simulink model "OpenFAST_ROSCO_FFP"  (R2021b)
settings: Solver=ode4  StartTime=0.0  StopTime=TMax  FixedStep=DT  MaxStep=DT  RelTol=1e-3  EnableMultiTasking=on
values from neighbouring files (symbols this model uses):
  P = ReadWrite_FAST(fast)    [RunExample_Simulink.m]
undefined symbols (not defined in the file or in its folder): F, GetFASTPar, OutList, R, simu, strmatch
libraries: simulink x1
settings Model: Creator=bjonkman  LastModifiedBy=david
settings SolverCC: AlgebraicLoopSolver=TrustRegion
settings DataIOCC: LimitDataPoints=on  SaveFormat=Array  SignalLoggingSaveFormat=ModelDataLogs  SaveOutput=off  SaveTime=off  ReturnWorkspaceOutputs=off  SignalLoggingName=sigsOut
settings OptimizationCC: ExpressionDepthLimit=2147483647  LifeSpan=inf
settings DebuggingCC: SaveWithParameterizedLinksMsg=none  UnderspecifiedInitializationDetection=Classic  MergeDetectMultiDrivingBlocksExec=none  SignalResolutionControl=TryResolveAllWithWarning  MultiTaskDSMMsg=warning  MultiTaskCondExecSysMsg=none  FcnCallInpInsideContextMsg=warning  StateNameClashWarn=warning  SFUnexpectedBacktrackingDiag=warning  SFNoUnconditionalDefaultTransitionDiag=warning  SFExecutionAtInitializationDiag=none  SFMachineParentedDataDiag=warning  ArithmeticOperatorsInVariantConditions=warning
settings HardwareCC: ProdBitPerPointer=32  ProdBitPerSizeT=32  ProdBitPerPtrDiffT=32  ProdLargestAtomicFloat=None  ProdIntDivRoundTo=Undefined  ProdEndianess=Unspecified  ProdWordSize=32  ProdHWDeviceType=32-bit Generic  TargetUnknown=on
settings ModelReferenceCC: PropagateSignalLabelsOutOfModel=off
settings SFSimCC: SimUseLocalCustomCode=off  CustomCodeUndefinedFunction=UseInterfaceOnly
settings RTWCC: RTWUseLocalCustomCode=off
settings CodeAppCC: StateflowObjectComments=on
settings GRTTargetCC: TargetLangStandard=C89/C90 (ANSI)  CombineOutputUpdateFcns=off  GRTInterface=on
settings ConfigComp: CovMetricSettings=dw  CovSaveCumulativeToWorkspaceVar=on  CovSaveSingleToWorkspaceVar=on  CovExternalEMLEnable=off

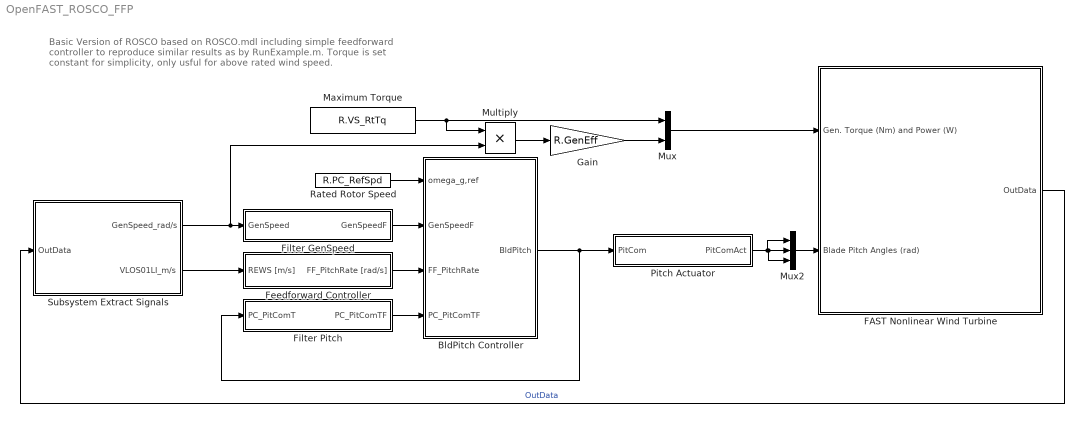
== system OpenFAST_ROSCO_FFP ==
  note: Basic Version of ROSCO based on ROSCO.mdl including simple feedforward controller to reproduce similar results as by RunExample.m.
      | Torque is set constant for simplicity, only usful for above rated wind speed.
  "  FAST Nonlinear Wind Turbine" : Subsystem  mask(FAST Nonlinear Wind Turbine){}
      mask help: This block contains the FAST S-Function.
      mask init:
      | clear FAST_SFunc
  BldPitch Controller : Subsystem
  Feedforward Controller : Subsystem
  Filter GenSpeed : Subsystem
  Filter Pitch : Subsystem
  Gain : Gain  Gain=R.GenEff
  Maximum Torque : Constant  Value=R.VS_RtTq
  Multiply : Product
  Mux : Mux  Inputs=2
  Mux2 : Mux  Inputs=3
  Pitch Actuator : Subsystem
  Rated Rotor Speed : Constant  Value=R.PC_RefSpd
  Subsystem Extract Signals : Subsystem
  wires:
  Mux2/1 -> "  FAST Nonlinear Wind Turbine"/2(Blade Pitch Angles (rad))
  BldPitch Controller/1(BldPitch) -> Filter Pitch/1(PC_PitComT), Pitch Actuator/1(PitCom)
  Rated Rotor Speed/1 -> BldPitch Controller/1(omega_g,ref)
  Subsystem Extract Signals/1(GenSpeed_rad/s) -> Multiply/2, Filter GenSpeed/1(GenSpeed)
  Maximum Torque/1 -> Mux/1, Multiply/1
  Filter GenSpeed/1(GenSpeedF) -> BldPitch Controller/2(GenSpeedF)
  Gain/1 -> Mux/2
  Mux/1 -> "  FAST Nonlinear Wind Turbine"/1(Gen. Torque (Nm) and Power (W))
  Multiply/1 -> Gain/1
  "  FAST Nonlinear Wind Turbine"/1(OutData) -> Subsystem Extract Signals/1(OutData)  "OutData"
  Filter Pitch/1(PC_PitComTF) -> BldPitch Controller/4(PC_PitComTF)
  Pitch Actuator/1(PitComAct) -> Mux2/1, Mux2/3, Mux2/2
  Feedforward Controller/1(FF_PitchRate [rad/s]) -> BldPitch Controller/3(FF_PitchRate)
  Subsystem Extract Signals/2(VLOS01LI_m/s) -> Feedforward Controller/1(REWS [m/s])

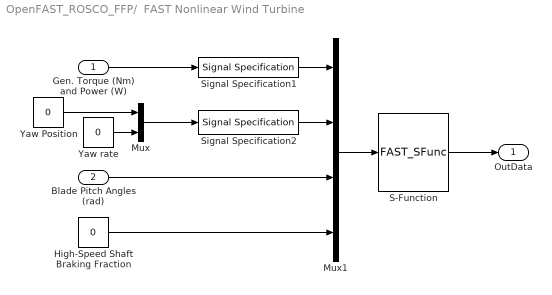
== system OpenFAST_ROSCO_FFP/  FAST Nonlinear Wind Turbine ==
  Gen. Torque (Nm) and Power (W) : Inport
  Blade Pitch Angles (rad) : Inport  Port=2
  High-Speed Shaft Braking Fraction : Constant  Value=0
  Mux : Mux  Inputs=2
  Mux1 : Mux
  S-Function : S-Function  FunctionName=FAST_SFunc  Parameters=FAST_InputFileName, TMax, 0  SFunctionDeploymentMode=off  EnableBusSupport=off
  Signal Specification1 : SignalSpecification  OutDataTypeStr=double  Dimensions=2
  Signal Specification2 : SignalSpecification  OutDataTypeStr=double  Dimensions=2
  Yaw Position : Constant  Value=0
  Yaw rate : Constant  Value=0
  OutData : Outport
  wires:
  Gen. Torque (Nm) and Power (W)/1 -> Signal Specification1/1
  S-Function/1 -> OutData/1
  Mux1/1 -> S-Function/1
  Blade Pitch Angles (rad)/1 -> Mux1/3
  Signal Specification1/1 -> Mux1/1
  Signal Specification2/1 -> Mux1/2
  High-Speed Shaft Braking Fraction/1 -> Mux1/4
  Yaw rate/1 -> Mux/2
  Mux/1 -> Signal Specification2/1
  Yaw Position/1 -> Mux/1

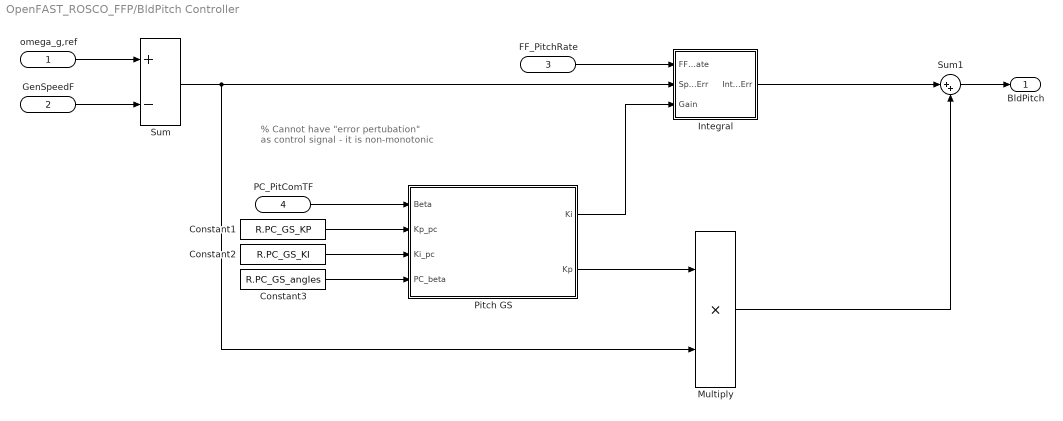
== system OpenFAST_ROSCO_FFP/BldPitch Controller ==
  note: % Cannot have "error pertubation" as control signal
      | - it is non-monotonic
  omega_g,ref : Inport
  GenSpeedF : Inport  Port=2
  FF_PitchRate : Inport  Port=3
  PC_PitComTF : Inport  Port=4
  Constant1 : Constant  Value=R.PC_GS_KP
  Constant2 : Constant  Value=R.PC_GS_KI
  Constant3 : Constant  Value=R.PC_GS_angles
  Integral : Subsystem
  Multiply : Product
  Pitch GS : MATLAB Function  TreatAsAtomicUnit=on
  Sum : Sum  Inputs=+-
  Sum1 : Sum  Inputs=|++
  BldPitch : Outport  VectorParamsAs1DForOutWhenUnconnected=off
  wires:
  Pitch GS/1(Ki) -> Integral/3(Gain)
  omega_g,ref/1 -> Sum/1
  GenSpeedF/1 -> Sum/2
  Constant1/1 -> Pitch GS/2(Kp_pc)
  Constant2/1 -> Pitch GS/3(Ki_pc)
  Constant3/1 -> Pitch GS/4(PC_beta)
  Sum/1 -> Multiply/2, Integral/2(SpeedErr)
  Multiply/1 -> Sum1/2
  Integral/1(IntSpdErr) -> Sum1/1
  Sum1/1 -> BldPitch/1
  PC_PitComTF/1 -> Pitch GS/1(Beta)
  FF_PitchRate/1 -> Integral/1(FF_PitchRate)
  Pitch GS/2(Kp) -> Multiply/1

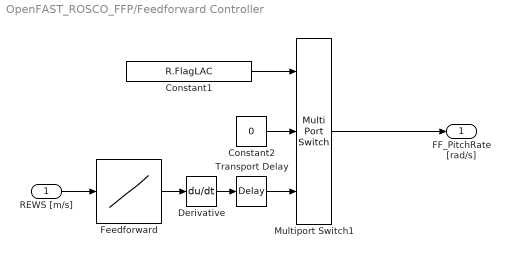
== system OpenFAST_ROSCO_FFP/Feedforward Controller ==
  REWS [m/s] : Inport
  Constant1 : Constant  Value=R.FlagLAC
  Constant2 : Constant  Value=0
  Derivative : Derivative
  Feedforward : Lookup_n-D  NumberOfTableDimensions=1  BreakpointsForDimension1=R.StaticWind  Table=R.StaticPitch  InternalRulePriority=Speed  RndMeth=Simplest  InputSameDT=on
  Multiport Switch1 : MultiPortSwitch  DataPortOrder=Specify indices  Inputs=2  DataPortIndices={0,1}
  Transport Delay : TransportDelay  DelayTime=R.T_buffer
  FF_PitchRate [rad/s] : Outport  VectorParamsAs1DForOutWhenUnconnected=off
  wires:
  Multiport Switch1/1 -> FF_PitchRate [rad/s]/1
  Feedforward/1 -> Derivative/1
  Derivative/1 -> Transport Delay/1
  Constant1/1 -> Multiport Switch1/1
  Constant2/1 -> Multiport Switch1/2
  REWS [m/s]/1 -> Feedforward/1
  Transport Delay/1 -> Multiport Switch1/3

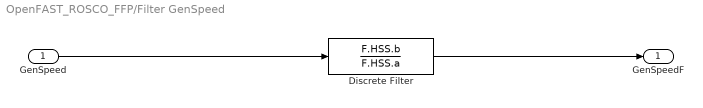
== system OpenFAST_ROSCO_FFP/Filter GenSpeed ==
  GenSpeed : Inport
  Discrete Filter : DiscreteFilter  Numerator=F.HSS.b  Denominator=F.HSS.a  InitialStates=R.PC_RefSpd/(sum(F.HSS.a(2:end))+1)
  GenSpeedF : Outport  VectorParamsAs1DForOutWhenUnconnected=off
  wires:
  Discrete Filter/1 -> GenSpeedF/1
  GenSpeed/1 -> Discrete Filter/1

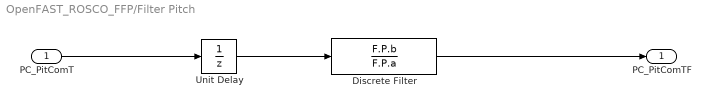
== system OpenFAST_ROSCO_FFP/Filter Pitch ==
  PC_PitComT : Inport
  Discrete Filter : DiscreteFilter  Numerator=F.P.b  Denominator=F.P.a
  Unit Delay : UnitDelay  SampleTime=-1  HasFrameUpgradeWarning=on
  PC_PitComTF : Outport  VectorParamsAs1DForOutWhenUnconnected=off
  wires:
  PC_PitComT/1 -> Unit Delay/1
  Discrete Filter/1 -> PC_PitComTF/1
  Unit Delay/1 -> Discrete Filter/1

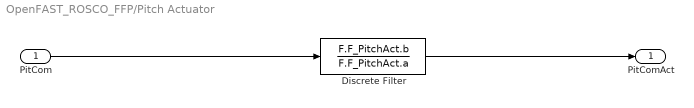
== system OpenFAST_ROSCO_FFP/Pitch Actuator ==
  PitCom : Inport
  Discrete Filter : DiscreteFilter  Numerator=F.F_PitchAct.b  Denominator=F.F_PitchAct.a  InitialStates=GetFASTPar(P.EDP,'BlPitch(1)')/180*pi/(sum(F.F_PitchAct.a(2:end))+1)
  PitComAct : Outport  VectorParamsAs1DForOutWhenUnconnected=off
  wires:
  PitCom/1 -> Discrete Filter/1
  Discrete Filter/1 -> PitComAct/1

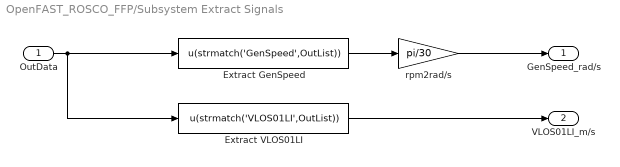
== system OpenFAST_ROSCO_FFP/Subsystem Extract Signals ==
  OutData : Inport
  Extract GenSpeed : Fcn  Expr=u(strmatch('GenSpeed',OutList))
  Extract VLOS01LI : Fcn  Expr=u(strmatch('VLOS01LI',OutList))
  rpm2rad/s : Gain  Gain=pi/30
  GenSpeed_rad/s : Outport  VectorParamsAs1DForOutWhenUnconnected=off
  VLOS01LI_m/s : Outport  Port=2  VectorParamsAs1DForOutWhenUnconnected=off
  wires:
  rpm2rad/s/1 -> GenSpeed_rad/s/1
  Extract GenSpeed/1 -> rpm2rad/s/1
  OutData/1 -> Extract GenSpeed/1, Extract VLOS01LI/1
  Extract VLOS01LI/1 -> VLOS01LI_m/s/1

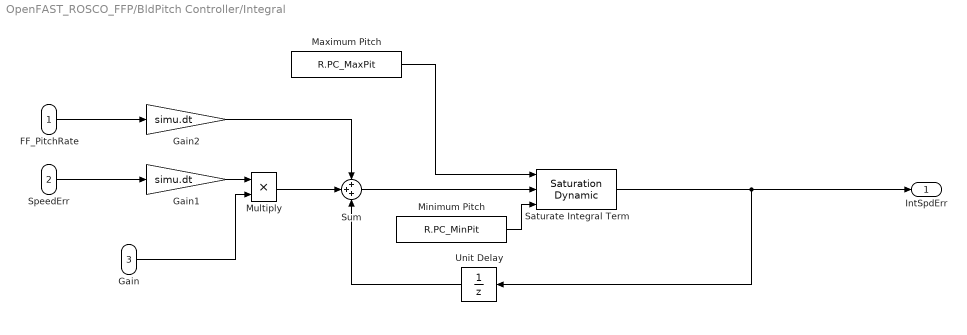
== system OpenFAST_ROSCO_FFP/BldPitch Controller/Integral ==
  FF_PitchRate : Inport
  SpeedErr : Inport  Port=2
  Gain : Inport  Port=3
  Gain1 : Gain  Gain=simu.dt
  Gain2 : Gain  Gain=simu.dt
  Maximum Pitch : Constant  Value=R.PC_MaxPit
  Minimum Pitch : Constant  Value=R.PC_MinPit
  Multiply : Product
  Saturate Integral Term : simulink/Discontinuities/Saturation Dynamic  OutMin=[]  OutMax=[]  OutDataTypeStr=Inherit: Same as second input  OutDataType=fixdt(1, 16)  OutScaling=2^-10  RndMeth=Nearest  DoSatur=off
  Sum : Sum  Inputs=+++
  Unit Delay : UnitDelay  InitialCondition=GetFASTPar(P.EDP,'BlPitch(1)')/180*pi  SampleTime=-1  HasFrameUpgradeWarning=on
  IntSpdErr : Outport  VectorParamsAs1DForOutWhenUnconnected=off
  wires:
  Maximum Pitch/1 -> Saturate Integral Term/1
  Sum/1 -> Saturate Integral Term/2
  SpeedErr/1 -> Gain1/1
  Gain/1 -> Multiply/2
  Saturate Integral Term/1 -> IntSpdErr/1, Unit Delay/1
  Gain1/1 -> Multiply/1
  Minimum Pitch/1 -> Saturate Integral Term/3
  Unit Delay/1 -> Sum/3
  Multiply/1 -> Sum/2
  Gain2/1 -> Sum/1
  FF_PitchRate/1 -> Gain2/1

== matlab function OpenFAST_ROSCO_FFP/BldPitch Controller/Pitch GS ==
  data: Ki output size=1; Beta input; Kp_pc input; Kp output size=1; Ki_pc input; PC_beta input
 function [Ki, Kp] = GainSchedule(Beta, Kp_pc, Ki_pc,  PC_beta)

% This function calculates the current gains for a Collective Blade Pitch 
% controller
%
% Inputs: v - Current wind speed estimate, m/s.
%         ContParam - Structure of control parameters, output from
%                     ControlParameters.m
%
% Outputs: Kp - Proportional Gain
%          Ki - Integral Gain
%
% Nikhar Abbas - May 2019


%% Linear Gain Schedule
% pKp_pc = ContParam.GS.pKp_pc;
% pKi_pc = ContParam.GS.pKi_pc;
% 
% %%
% Kp = pKp_pc(1)*Beta + pKp_pc(2);
% Ki = pKi_pc(1)*Beta + pKi_pc(2);
% % Kp = pKp_pc(1)*v + pKp_pc(2)
% % Ki = pKi_pc(1)*v + pKi_pc(2);
% 
% Kpmax = pKp_pc(1)*15*pi/180 + pKp_pc(2);
% Kimax = pKi_pc(1)*15*pi/180 + pKi_pc(2);
% 
% Kp = min(Kp, Kpmax);
% Ki = min(Ki,Kimax);

%% nonlinear Gain Schedule
% Kp_pc   = R.PC_GS_KP;
% Ki_pc   = R.PC_GS_KI;
% PC_beta = R.PC_GS_angles;

beta    = max(min(Beta,PC_beta(end)), PC_beta(1));

% gains
Kp      = interp1(PC_beta,Kp_pc, beta);
Ki      = interp1(PC_beta,Ki_pc, beta);



end
